simulink model "System2"  (R2023a)
settings: Solver=ode113  StartTime=0.0  StopTime=inf  MinStep=1  RelTol=1e-3
libraries: simulink x3783, slpidlib x2
(part 158 of 158)

== system System2/Battery2/Module2/SubModule_2/Cell9/2RC/RC2 ==
  Current : Inport
  R : Inport  Port=2
  C : Inport  Port=3
  2 : Constant
  Add : Sum
  Divide : Product  Inputs=*/
  Divide1 : Product  Inputs=*/
  Divide2 : Product  Inputs=/*
  Divide3 : Product  Inputs=**
  Integrator1 : Integrator
  Integrator2 : Integrator
  V : Outport
  wires:
  C/1 -> Divide2/1, Divide1/2
  Integrator1/1 -> Divide/1
  Divide1/1 -> Integrator1/1
  Add/1 -> Divide/2
  R/1 -> Add/1, Divide1/1
  Divide2/1 -> Integrator2/1
  Divide/1 -> Divide3/2
  Current/1 -> Divide3/1
  Divide3/1 -> V/1
  Integrator2/1 -> Add/2
  2/1 -> Divide2/2

== system System2/Battery2/Module2/SubModule_2/Cell9/2RC/Rint ==
  Current : Inport
  R : Inport  Port=2
  Divide3 : Product  Inputs=**
  V : Outport
  wires:
  Divide3/1 -> V/1
  Current/1 -> Divide3/1
  R/1 -> Divide3/2

== system System2/Battery2/Module2/SubModule_2/Cell9/SOCEstimator/SOCEstimator ==
  SOC_Initial : Inport
  Current : Inport  Port=2
  CellCapacity : Inport  Port=3
  Add1 : Sum  Inputs=+-
  Constant : Constant  Value=100  SampleTime=-1
  Constant1 : Constant  Value=3600  SampleTime=-1
  Delay : Delay  DelayLength=1  InitialConditionSource=Input port
      settings: InputPortMap=u0,p4
  Divide : Product  Inputs=*//
  Divide1 : Product  Inputs=*/
  Integrator : Integrator
  Saturation1 : Saturate  UpperLimit=1  LowerLimit=0
  SOC : Outport
  wires:
  Integrator/1 -> Divide/1
  Constant1/1 -> Divide/3
  CellCapacity/1 -> Divide/2
  Delay/1 -> SOC/1
  Current/1 -> Integrator/1
  SOC_Initial/1 -> Divide1/1
  Saturation1/1 -> Delay/1
  Divide/1 -> Add1/2
  Divide1/1 -> Add1/1, Delay/2
  Constant/1 -> Divide1/2
  Add1/1 -> Saturation1/1

== matlab function System2/Load_Split ==
  data: I_Load input; I_Battery1 output; I_Battery2 output; factor input; Max_I_Battery1 input; I_Battery2_act input
function [I_Battery1, I_Battery2] = Load_Split(I_Load,factor,Max_I_Battery1,I_Battery2_act)   % This is a more explicit version to satisfy the code analyzer. \n   % Define a constant for pi. \n  
I_Battery1 = 0;
I_Battery2 = 0;
if abs(I_Load) < factor*Max_I_Battery1
    I_Battery1 = I_Load;
    I_Battery2 = 0;
elseif I_Load > 0
    I_Battery2 = I_Load - factor*Max_I_Battery1;
    %I_Battery1 = factor*Max_I_Battery1;
    I_Battery1 = I_Load - I_Battery2_act;
elseif I_Load < 0
    I_Battery2 = I_Load + factor*Max_I_Battery1;
    %I_Battery1 = -factor*Max_I_Battery1;
    I_Battery1 = I_Load - I_Battery2_act;
end

== matlab function System2/DAB_Converter/DAB_Power_Eqn ==
  data: V1 input; P output; V2 input; phi input; n input; f input; L input
function P = dab_power(V1, V2, phi, n, f, L)   % This is a more explicit version to satisfy the code analyzer. \n   % Define a constant for pi. \n   
PI_CONST = 3.1415926535;  % Calculate the main gain term. \n   
K = (n * V1 * V2) / (2 * PI_CONST * f * L); % Calculate the term dependent on the phase shift. \n   
phi_term = phi * (1 - abs(phi)/PI_CONST); % Assign the final output. \n  
P = K * phi_term;

== matlab function System2/Load/MATLAB Function ==
  data: Torque input; Quadrant output; Speed input
function Quadrant = Quadrant_Selector(Torque,Speed)
if (Torque*Speed) < 0
    Quadrant = 0;
else
    Quadrant = 1;
end
